simulink model "Vector_FFT_Float_Ex2"  (R2025a)
settings: Solver=ode45  StartTime=0.0  StopTime=2048/10e3  RelTol=1e-3  EnableMultiTasking=on
undefined symbols (not defined in the file): S, vsva2785, xcvp1552
libraries: hdlSSR x5, hdlBasic x2, dspsrcs4 x1, dspxfrm3 x1, vmcUtilities x1
settings Model: Creator=dahlawat  LastModifiedBy=robg
settings SolverCC: AlgebraicLoopSolver=TrustRegion
settings DataIOCC: LimitDataPoints=on  SaveFormat=Array  ReturnWorkspaceOutputs=off
settings OptimizationCC: LifeSpan=inf
settings DebuggingCC: UnderspecifiedInitializationDetection=Classic  MergeDetectMultiDrivingBlocksExec=none  SolverPrmCheckMsg=warning  UnconnectedInputMsg=warning  UnconnectedOutputMsg=warning  UnconnectedLineMsg=warning  StateNameClashWarn=warning  SFUnexpectedBacktrackingDiag=warning  SFNoUnconditionalDefaultTransitionDiag=warning  SFExecutionAtInitializationDiag=none  ArithmeticOperatorsInVariantConditions=warning
settings HardwareCC: ProdBitPerPointer=32.0  ProdBitPerSizeT=32.0  ProdBitPerPtrDiffT=32.0  ProdLargestAtomicFloat=None  ProdIntDivRoundTo=Undefined  ProdEndianess=Unspecified  ProdWordSize=32.0  ProdHWDeviceType=32-bit Generic
settings ModelReferenceCC: EnableRefExpFcnMdlSchedulingChecks=on  PropagateSignalLabelsOutOfModel=off
settings SFSimCC: SimUseLocalCustomCode=off  CustomCodeUndefinedFunction=UseInterfaceOnly
settings RTWCC: RTWUseLocalCustomCode=off  GPUComputeCapability=3.5  DLArmComputeVersion=19.05
settings CodeAppCC: StateflowObjectComments=on
settings GRTTargetCC: TargetLangStandard=C89/C90 (ANSI)
settings ConfigComp: CovMetricSettings=dw  CovSaveCumulativeToWorkspaceVar=on  CovSaveSingleToWorkspaceVar=on  CovExternalEMLEnable=off

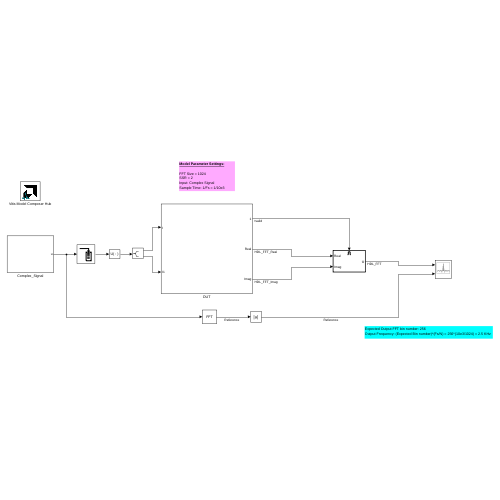
[thumbnail: Simulink's stored preview of the top-level diagram]
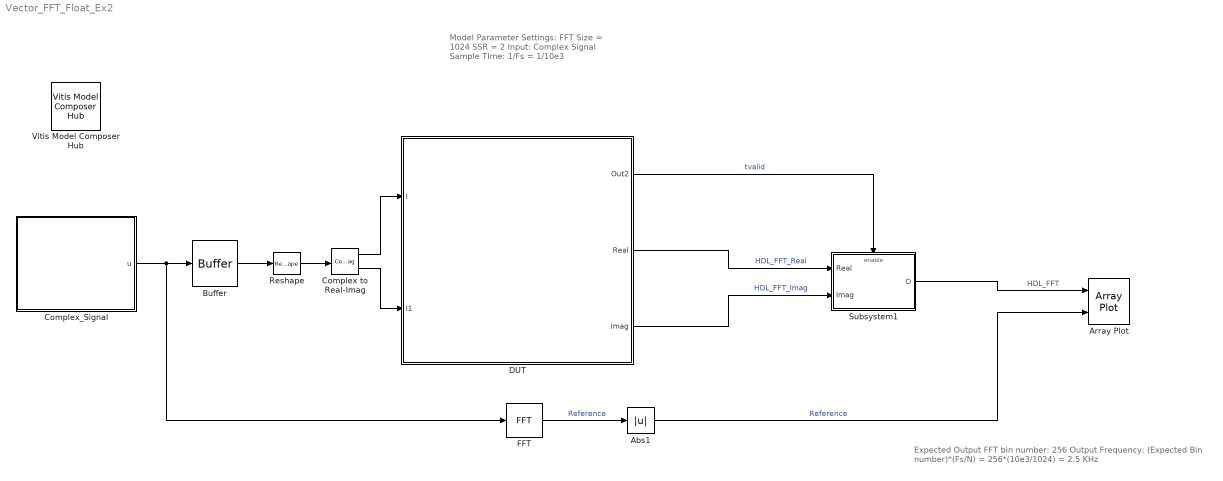
== system Vector_FFT_Float_Ex2 ==
  note: Expected Output FFT bin number: 256
      | Output Frequency: (Expected Bin number)*(Fs/N) = 256*(10e3/1024) = 2.5 KHz
  note: Model Parameter Settings:
      |
      | FFT Size = 1024
      | SSR = 2
      | Input: Complex Signal
      | Sample TIme: 1/Fs = 1/10e3
  Abs1 : Abs  SaturateOnIntegerOverflow=off
  Array Plot : ArrayPlot  NumInputPorts=2  WindowPosition=[1.000000,1.000000,1920.000000,1149.000000,]  Visible=on  ScopeFrameLocation=window  PlotType=Line  YLimits=[-2.3479 24.476]  ShowLegend=on
  Buffer : Buffer  N=2  OutputFrames=off
  Complex to Real-Imag : ComplexToRealImag
  Complex_Signal : Subsystem
  DUT : Subsystem
  FFT : dspxfrm3/FFT  FFTImplementation=Auto  CompMethod=Table lookup  TableOpt=NEW  TableOptActive=Speed  BitRevOrder=off  Normalize=off  InheritFFTLength=on  FFTLength=64  WrapInput=on  roundingMode=Ceiling  overflowMode=off  firstCoeffDataTypeStr=Inherit: Same word length as input  firstCoeffLastDataTypeStr=Inherit: Same word length as input  outputMin=[]  outputMax=[]
  Reshape : Reshape
  Subsystem1 : Subsystem
  Vitis Model Composer Hub : vmcUtilities/Vitis Model Composer Hub  Tag=genX  CodeGeneration=off  SubsystemName=DUT  CompilationType=HDLCompilation  SubsystemType=HDLNode  ExportTypeV2=IP Catalog  StartColumn=1  NumberOfColumns=1  TargetDirectory=./netlist  exportDesign=off  analyzeDesign=on  validateDesignOnHw=off  ExportType=HW Code  IpVendor=xilinx.com  IpLibrary=hls  IpVersion=1.0  IpHWLanguage=Verilog  AieCompilerOptions={}  AieSimulatorOptions={}  CreateTestbench=on  TestbenchStackSize=10  RunRtlSim=off  RunCSim=off  RunAieSim=on  enableSimulationTimeout=on  enableGraphIterations=on  AieSimTimeout=50000  AieGraphIterations=-1  RunAieSimProfiling=off  LaunchVitisAnalyzer=off  PlotOutput=off  RunX86Sim=off  X86SimTimeout=10  GenHwImage=off  GenLibadfXo=on  GenHwValidationCode=off  PlatformType=Not Specified  HwSystemType=Baremetal  HwValidationTarget=hw  ProjDevice=xcvp1552-vsva2785-1LP-e-S  ProjDevicePart=xcvp1552-vsva2785-1LP-e-S  AIEType=None  SamplePeriod=-1  ClockFrequency=200  DataPathParallelism=1  xilinxfamily=versalpremium  part=xcvp1552  speed=-1LP-e-S  package=vsva2785  directory=./netlist/ip/DUT/src  testbench=off  incr_netlist=off  synthesis_tool=Vivado  clock_wrapper=Clock Enables  dbl_ovrd=According to Block Masks  dcm_input_clock_period=10  sysclk_period=10  simulink_period=1/10e3  eval_field=0  IPInfoJsonString="{\"DUTSubsystemName\":\"Vector_IFFT_FLOAT\",\"HDLSubsystem\":{\"SubsystemName\":\"Vector_IFFT_FLOAT\",\"IPName\":\"Vector_IFFT_FLOAT\",\"IPLibrary\":\"VMC\",\"IPVendor\":\"User Company\",\"IPVersion\":\"1.0\",\"TargetDirectory\":\"./netlist\",\"SubsystemDir\":\"./netlist/ip/Vector_IFFT_FLOAT\",\"FreqHz\":\"100000000\"},\"SubsystemTag\":\"HDLNode\"}"  LogFileName=/proj/xhdhdstaff5/sdegala/Head1/HEAD/2025_1_newBlocks/netlist/model_composer.log  NThreads=4  IPConfigFile=/tmp/vmctmp-sdegala/1167582/ipconfig.json
  wires:
  Complex_Signal/1(u) -> FFT/1, Buffer/1
  DUT/1(Out2) -> Subsystem1/Enable  "tvalid"
  FFT/1 -> Abs1/1  "Reference"
  Buffer/1 -> Reshape/1
  Reshape/1 -> Complex to Real-Imag/1
  Complex to Real-Imag/1 -> DUT/1(I)
  Complex to Real-Imag/2 -> DUT/2(I1)
  DUT/2(Real) -> Subsystem1/1(Real)  "HDL_FFT_Real"
  DUT/3(Imag) -> Subsystem1/2(Imag)  "HDL_FFT_Imag"
  Abs1/1 -> Array Plot/2  "Reference"
  Subsystem1/1(O) -> Array Plot/1  "HDL_FFT"

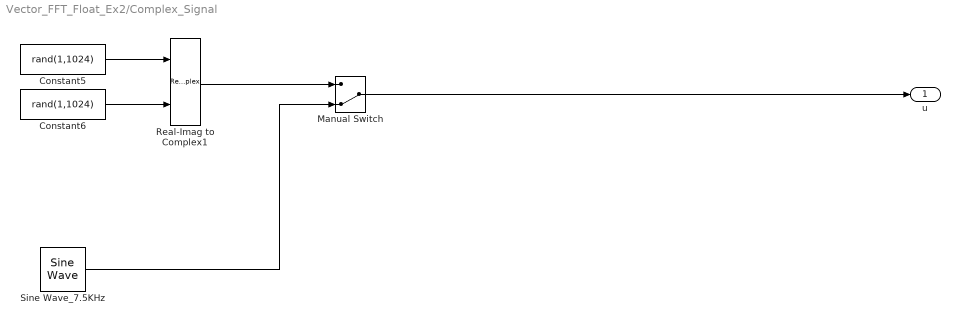
== system Vector_FFT_Float_Ex2/Complex_Signal ==
  Constant5 : Constant  Value=rand(1,1024)  OutDataTypeStr=single  SampleTime=-1
  Constant6 : Constant  Value=rand(1,1024)  OutDataTypeStr=single  SampleTime=-1
  Manual Switch : ManualSwitch  CurrentSetting=0
  Real-Imag to Complex1 : RealImagToComplex
  Sine Wave_7.5KHz : dspsrcs4/Sine Wave  Amplitude=1  Frequency=2.5e3  Phase=0  SampleMode=Discrete  OutComplex=Complex  CompMethod=Trigonometric fcn  TableSize=Speed  SampleTime=1/10e3  SamplesPerFrame=1024  ResetState=Restart at time zero  OutputFrames=off  dataType=single  wordLen=16  udDataType=sfix(16)  fracBitsMode=Best precision  numFracBits=15  OutDataTypeStr=single  LastOutDataTypeStr=single
  u : Outport
  wires:
  Constant5/1 -> Real-Imag to Complex1/1
  Constant6/1 -> Real-Imag to Complex1/2
  Real-Imag to Complex1/1 -> Manual Switch/1
  Sine Wave_7.5KHz/1 -> Manual Switch/2
  Manual Switch/1 -> u/1

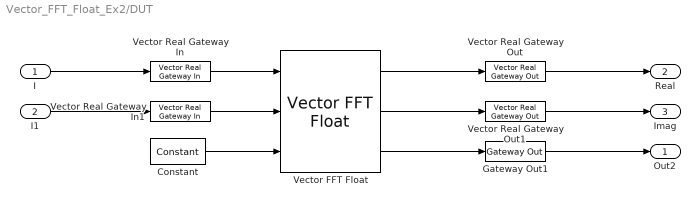
== system Vector_FFT_Float_Ex2/DUT ==
  I : Inport
  I1 : Inport  Port=2
  Constant : hdlBasic/Constant  const=1.0  gui_display_data_type=Boolean  arith_type=Boolean  n_bits=16  bin_pt=14  preci_type=Single  exp_width=8  frac_width=24  explicit_period=on  period=1/10e3  XmcBlockStatus=1  maskContainerNames=tabcontainer1  block_type=constant  block_config=sysgen:Constant_config
  Gateway Out1 : hdlBasic/Gateway Out  inherit_from_input=off  bool_to_boolean=off  hdl_port=on  rows=1  columns=1  UseAsDAC=off  DACChannel='1'  interface=None  automatic_assignment=on  address_offset=hex2dec('00')  intf_name=''  intf_description=''  timing_constraint=None  locs_specified=off  LOCs={}  io_standard={}  XmcBlockStatus=1  maskContainerNames=group4  block_type=gatewayout  block_config=sysgen:gateway_out_config  block_width_w=590  block_height_w=620  block_width=620  block_height=750
  Vector FFT Float : hdlSSR/Vector FFT Float  N=1024  sg_ssr=2  bram_threshold=258  block_type=fft_float_ssr  ox=-1000  oy=-1000  use_cb=on  XmcBlockStatus=1  sg_ssr_prev=2  maskContainerNames=group3
  Vector Real Gateway In : hdlSSR/Vector Real Gateway In  gui_display_data_type=Floating-point  arith_type=Floating-point  n_bits=16  bin_pt=14  preci_type=Single  exp_width=8  frac_width=24  quantization="Round  (unbiased: +/- Inf)"  overflow=Saturate  period=1/10e3  sg_ssr=2  UseAsADC=off  ADCChannel='1'  interface=None  automatic_assignment=on  address_offset=hex2dec('00')  intf_name=''  intf_description=''  default_value=0  timing_constraint=None  locs_specified=off  LOCs={}  io_standard={}  inherit_from_input=off  hdl_port=on  interface_prev=1  block_type=realgatewayin_ssr  XmcBlockStatus=1  sg_ssr_prev=2  maskContainerNames=group4  block_width_w=590  block_height_w=670  block_width=640  block_height=850
  Vector Real Gateway In1 : hdlSSR/Vector Real Gateway In  gui_display_data_type=Floating-point  arith_type=Floating-point  n_bits=16  bin_pt=14  preci_type=Single  exp_width=8  frac_width=24  quantization="Round  (unbiased: +/- Inf)"  overflow=Saturate  period=1/10e3  sg_ssr=2  UseAsADC=off  ADCChannel='1'  interface=None  automatic_assignment=on  address_offset=hex2dec('00')  intf_name=''  intf_description=''  default_value=0  timing_constraint=None  locs_specified=off  LOCs={}  io_standard={}  inherit_from_input=off  hdl_port=on  interface_prev=1  block_type=realgatewayin_ssr  XmcBlockStatus=1  sg_ssr_prev=2  maskContainerNames=group4  block_width_w=590  block_height_w=670  block_width=640  block_height=850
  Vector Real Gateway Out : hdlSSR/Vector Real Gateway Out  inherit_from_input=on  hdl_port=on  sg_ssr=2  rows=1  columns=1  UseAsDAC=off  DACChannel='1'  interface=None  automatic_assignment=on  address_offset=hex2dec('00')  intf_name=''  intf_description=''  timing_constraint=None  locs_specified=off  LOCs={}  io_standard={}  block_type=realgatewayout_ssr  XmcBlockStatus=1  sg_ssr_prev=2  maskContainerNames=group4  block_width_w=590  block_height_w=620  block_width=620  block_height=750
  Vector Real Gateway Out1 : hdlSSR/Vector Real Gateway Out  inherit_from_input=on  hdl_port=on  sg_ssr=2  rows=1  columns=1  UseAsDAC=off  DACChannel='1'  interface=None  automatic_assignment=on  address_offset=hex2dec('00')  intf_name=''  intf_description=''  timing_constraint=None  locs_specified=off  LOCs={}  io_standard={}  block_type=realgatewayout_ssr  XmcBlockStatus=1  sg_ssr_prev=2  maskContainerNames=group4  block_width_w=590  block_height_w=620  block_width=620  block_height=750
  Out2 : Outport
  Real : Outport  Port=2
  Imag : Outport  Port=3
  wires:
  Constant/1 -> Vector FFT Float/3
  I/1 -> Vector Real Gateway In/1
  Vector Real Gateway Out/1 -> Real/1
  Vector FFT Float/3 -> Gateway Out1/1
  Gateway Out1/1 -> Out2/1
  I1/1 -> Vector Real Gateway In1/1
  Vector Real Gateway Out1/1 -> Imag/1
  Vector FFT Float/1 -> Vector Real Gateway Out/1
  Vector FFT Float/2 -> Vector Real Gateway Out1/1
  Vector Real Gateway In/1 -> Vector FFT Float/1
  Vector Real Gateway In1/1 -> Vector FFT Float/2

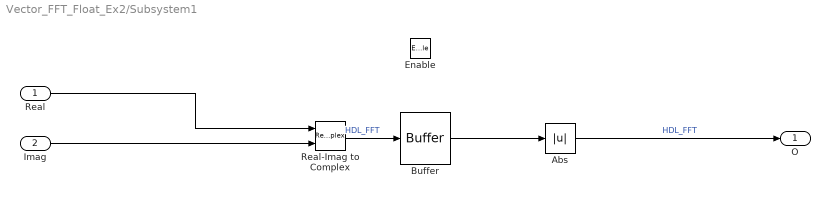
== system Vector_FFT_Float_Ex2/Subsystem1 ==
  Real : Inport
  Imag : Inport  Port=2
  Enable : EnablePort
  Abs : Abs  SaturateOnIntegerOverflow=off
  Buffer : Buffer  N=1024  OutputFrames=off
  Real-Imag to Complex : RealImagToComplex
  O : Outport
  wires:
  Buffer/1 -> Abs/1
  Abs/1 -> O/1  "HDL_FFT"
  Real-Imag to Complex/1 -> Buffer/1  "HDL_FFT"
  Imag/1 -> Real-Imag to Complex/2
  Real/1 -> Real-Imag to Complex/1
